simulink model "delay"  (R2019b)
settings: Solver=FixedStepAuto  StartTime=0.0  StopTime=10.0  FixedStep=T  RelTol=1e-3  EnableMultiTasking=on
undefined symbols (not defined in the file): A
libraries: arduinolib x1
settings Model: SimulationMode=external  SILPILModeSetting=veronly  ExtModeTrigDuration=2  Creator=Tyler  LastModifiedBy=Tyler
settings DataIOCC: InspectSignalLogs=on  LoggingToFile=on
settings OptimizationCC: GainParamInheritBuiltInType=on  UseFloatMulNetSlope=on  EnhancedBackFolding=on  PassReuseOutputArgsAs=Individual arguments  ZeroExternalMemoryAtStartup=off  ZeroInternalMemoryAtStartup=off  MaxStackSize=64  OptimizeBlockOrder=speed  DifferentSizesBufferReuse=on  OptimizationCustomize=off  EfficientTunableParamExpr=on
settings DebuggingCC: ParameterTunabilityLossMsg=error  SFUnexpectedBacktrackingDiag=warning  SFNoUnconditionalDefaultTransitionDiag=warning
settings HardwareCC: ProdBitPerInt=16  ProdBitPerPointer=16  ProdBitPerSizeT=16  ProdBitPerPtrDiffT=16  ProdLargestAtomicFloat=None  ProdWordSize=8  ProdHWDeviceType=Atmel->AVR
settings SFSimCC: MATLABDynamicMemAlloc=off
settings RTWCC: SystemTargetFile=ert.tlc  HardwareBoard=Arduino Nano 3.0  TLCOptions=-aInlineSetEventsForThisBaseRateFcn=TLC_FALSE -aSuppressMultiTaskScheduler=TLC_FALSE -aRateBasedStepFcn=1  TemplateMakefile=ert_default_tmf  GenerateReport=on  Toolchain=Arduino AVR  BuildConfiguration=Faster Runs  IncludeHyperlinkInReport=on  GenerateTraceInfo=on  GenerateTraceReport=on  GenerateTraceReportSl=on  GenerateTraceReportSf=on  GenerateTraceReportEml=on
settings CodeAppCC: ForceParamTrailComments=on  IgnoreCustomStorageClasses=off  OperatorAnnotations=on  SimulinkDataObjDesc=on  SFDataObjDesc=on  InsertBlockDesc=on  EnableCustomComments=on
settings ERTTargetCC: SupportContinuousTime=on  SupportVariableSizeSignals=on  ExtModeStaticAllocSize=250  RootIOFormat=Structure reference

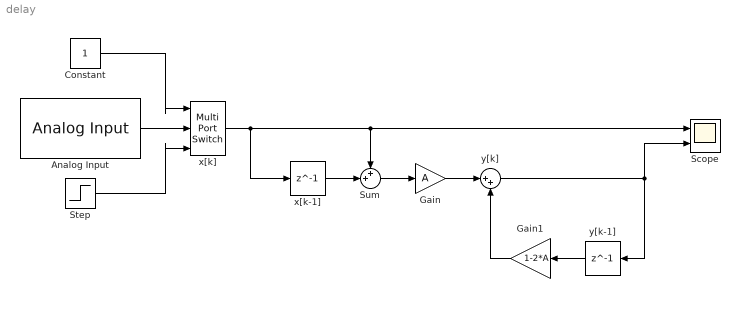
== system delay ==
  Analog Input : arduinolib/Analog Input  pinNumber=1  ReadResultsOnly=off  ConversionTriggerSource=Software  ExternalTriggerType=uint32(0)  OutputDataType=uint16  EnableConversionCompleteNotify=off  EnableOuputStatus=off  SampleTime=-1  blockPlatform=arduino
  Constant : Constant
  Gain : Gain  Gain=A
  Gain1 : Gain  Gain=1-2*A
  Scope : Scope  NumInputPorts=2
  Step : Step  SampleTime=0
  Sum : Sum  Inputs=++|
  x[k-1] : Delay  DelayLength=1
  x[k] : MultiPortSwitch  Inputs=2
  y[k-1] : Delay  DelayLength=1
  y[k] : Sum  Inputs=|++
  wires:
  x[k-1]/1 -> Sum/2
  Sum/1 -> Gain/1
  Gain/1 -> y[k]/1
  y[k]/1 -> y[k-1]/1, Scope/2
  y[k-1]/1 -> Gain1/1
  Gain1/1 -> y[k]/2
  x[k]/1 -> x[k-1]/1, Sum/1, Scope/1
  Step/1 -> x[k]/3
  Analog Input/1 -> x[k]/2
  Constant/1 -> x[k]/1
